simulink model "feedforward"  (R2016b)
settings: Solver=VariableStepAuto  StartTime=0.0  StopTime=48*60  RelTol=1e-3
values from neighbouring files (symbols this model uses):
  Ki = -0.075    [defineparams.m]    (also in smithpredictor_1.m)
  Km = 4    [defineparams.m]    (also in smithpredictor_1.m)
  s_den_c = double(coeffs(C_simple_den))    [Qdesign.m]
  s_num_c = double(coeffs(C_simple_num))    [Qdesign.m]
  Tdi = 25    [defineparams.m]    (also in smithpredictor_1.m)
  Tdm = 15    [defineparams.m]    (also in smithpredictor_1.m)
  Ti = 140    [defineparams.m]    (also in smithpredictor_1.m)
  Tm = 50    [defineparams.m]    (also in smithpredictor_1.m)
settings Model: Creator=Matt Cordoba  LastModifiedBy=Matt Cordoba

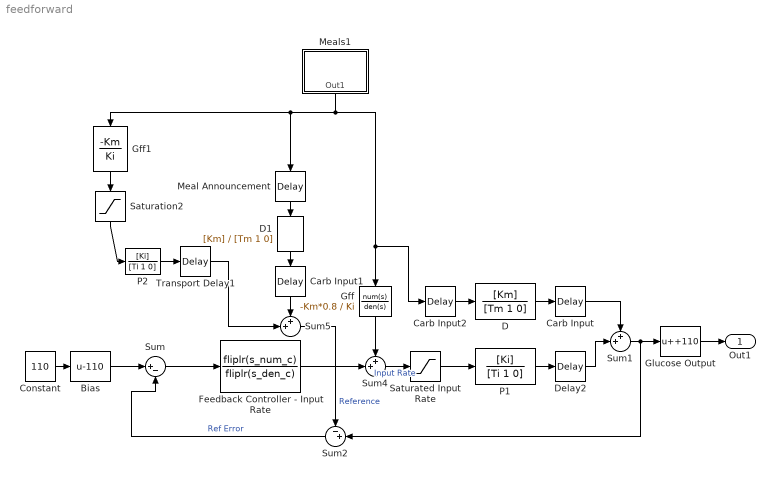
== system feedforward ==
  Bias : Bias  Bias=-110
  Carb Input : TransportDelay  DelayTime=Tdm
  Carb Input1 : TransportDelay  DelayTime=Tdm
  Carb Input2 : TransportDelay  DelayTime=10
  Constant : Constant  Value=110
  D : TransferFcn  Numerator=[Km]  Denominator=[Tm 1 0]
  D1 : TransferFcn  Numerator=[Km]  Denominator=[Tm 1 0]
  Delay2 : TransportDelay  DelayTime=Tdi
  Feedback Controller - Input Rate : TransferFcn  Numerator=fliplr(s_num_c)  Denominator=fliplr(s_den_c)
  Gff : TransferFcn  Numerator=-Km*0.8  Denominator=Ki
  Gff1 : TransferFcn  Numerator=-Km  Denominator=Ki
  Glucose Output : Bias  Bias=+110
  Meal Announcement : TransportDelay  DelayTime=10
  Meals1 : Subsystem
  P1 : TransferFcn  Numerator=[Ki]  Denominator=[Ti 1 0]
  P2 : TransferFcn  Numerator=[Ki]  Denominator=[Ti 1 0]
  Saturated Input Rate : Saturate  UpperLimit=166  LowerLimit=0
  Saturation2 : Saturate  UpperLimit=166  LowerLimit=0
  Sum : Sum  Inputs=|+-
  Sum1 : Sum  Inputs=++|
  Sum2 : Sum  Inputs=-+|
  Sum4 : Sum  Inputs=++|
  Sum5 : Sum  Inputs=++|
  Transport Delay1 : TransportDelay  DelayTime=Tdi
  Out1 : Outport
  wires:
  D/1 -> Carb Input/1
  Carb Input/1 -> Sum1/1
  P1/1 -> Delay2/1
  Delay2/1 -> Sum1/2
  Meals1/1(Out1) -> Carb Input2/1, Gff/1, Meal Announcement/1, Gff1/1
  Constant/1 -> Bias/1
  Bias/1 -> Sum/1
  Glucose Output/1 -> Out1/1
  Sum/1 -> Feedback Controller - Input Rate/1
  Feedback Controller - Input Rate/1 -> Sum4/2
  Gff/1 -> Sum4/1
  D1/1 -> Carb Input1/1
  Carb Input1/1 -> Sum5/1
  Gff1/1 -> Saturation2/1
  Saturation2/1 -> P2/1
  P2/1 -> Transport Delay1/1
  Transport Delay1/1 -> Sum5/2
  Sum1/1 -> Sum2/2, Glucose Output/1
  Carb Input2/1 -> D/1
  Meal Announcement/1 -> D1/1
  Sum2/1 -> Sum/2  "Ref Error"
  Sum4/1 -> Saturated Input Rate/1  "Input Rate"
  Sum5/1 -> Sum2/1  "Reference"
  Saturated Input Rate/1 -> P1/1

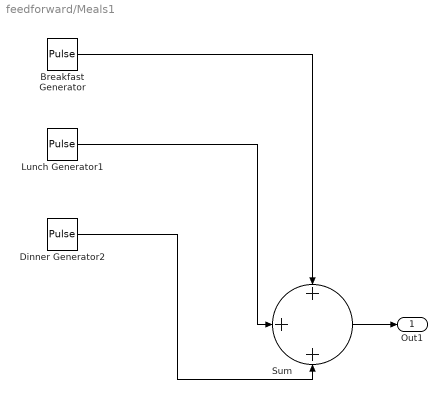
== system feedforward/Meals1 ==
  Breakfast Generator : DiscretePulseGenerator  Amplitude=25/10*1.25  Period=1440  PulseWidth=10  PhaseDelay=60
  Dinner Generator2 : DiscretePulseGenerator  Amplitude=3  Period=1440  PulseWidth=20  PhaseDelay=720
  Lunch Generator1 : DiscretePulseGenerator  Amplitude=40/15*1.25  Period=1440  PulseWidth=15  PhaseDelay=420
  Sum : Sum  Inputs=+++
  Out1 : Outport
  wires:
  Breakfast Generator/1 -> Sum/1
  Lunch Generator1/1 -> Sum/2
  Dinner Generator2/1 -> Sum/3
  Sum/1 -> Out1/1
